simulink model "nosaturation"  (R2016b)
settings: Solver=VariableStepAuto  StartTime=0.0  StopTime=48*60  RelTol=1e-3
values from neighbouring files (symbols this model uses):
  d1 = i_den(1)    [Qdesign.m]    (also in Qdesign2.m)
  d2 = i_den(2)    [Qdesign.m]    (also in Qdesign2.m)
  d3 = i_den(3)    [Qdesign.m]    (also in Qdesign2.m)
  d4 = i_den(4)    [Qdesign.m]    (also in Qdesign2.m)
  Ki = -0.075    [defineparams.m]    (also in smithpredictor_1.m)
  Km = 4    [defineparams.m]    (also in smithpredictor_1.m)
  n1 = 0    [Qdesign.m]    (also in Qdesign2.m)
  n2 = i_num(1)    [Qdesign.m]    (also in Qdesign2.m)
  n3 = i_num(2)    [Qdesign.m]    (also in Qdesign2.m)
  n4 = i_num(3)    [Qdesign.m]    (also in Qdesign2.m)
  s_den = double(coeffs(Q_simple_den))    [Qdesign.m]    (also in Qdesign2.m)
  s_num = [0 double(coeffs(Q_simple_num))]    [Qdesign.m]    (also in Qdesign2.m)
  Tdi = 25    [defineparams.m]    (also in smithpredictor_1.m)
  Tdm = 15    [defineparams.m]    (also in smithpredictor_1.m)
  Ti = 140    [defineparams.m]    (also in smithpredictor_1.m)
  Tm = 50    [defineparams.m]    (also in smithpredictor_1.m)
settings Model: Creator=Matt Cordoba  LastModifiedBy=Matt Cordoba

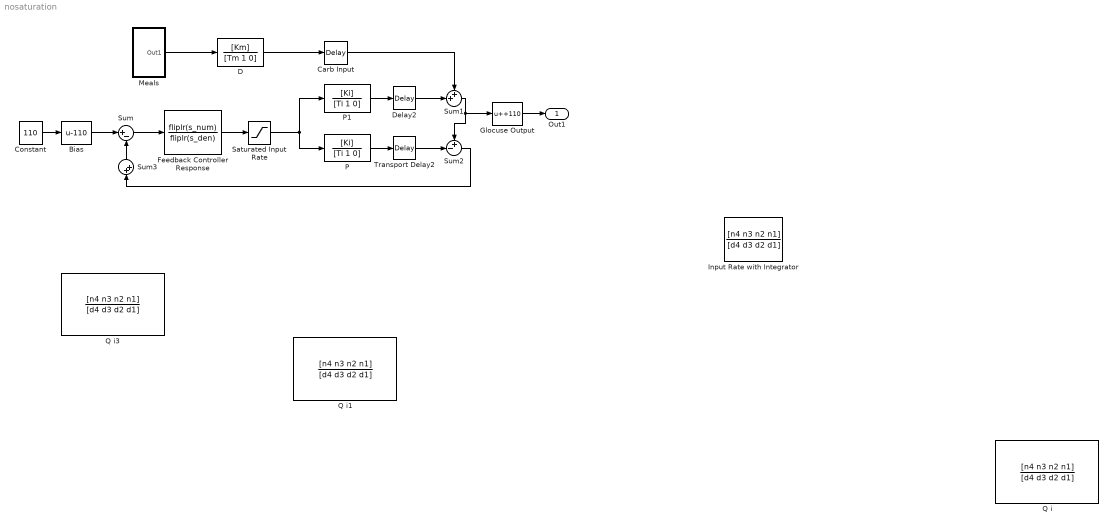
== system nosaturation ==
  Bias : Bias  Bias=-110
  Carb Input : TransportDelay  DelayTime=Tdm
  Constant : Constant  Value=110
  D : TransferFcn  Numerator=[Km]  Denominator=[Tm 1 0]
  Delay2 : TransportDelay  DelayTime=Tdi
  Feedback Controller Response : TransferFcn  Numerator=fliplr(s_num)  Denominator=fliplr(s_den)
  Glocuse Output : Bias  Bias=+110
  Input Rate with Integrator : TransferFcn  Numerator=[n4 n3 n2 n1]  Denominator=[d4 d3 d2 d1]
  Meals : Subsystem
  P : TransferFcn  Numerator=[Ki]  Denominator=[Ti 1 0]
  P1 : TransferFcn  Numerator=[Ki]  Denominator=[Ti 1 0]
  Q i : TransferFcn  Numerator=[n4 n3 n2 n1]  Denominator=[d4 d3 d2 d1]
  Q i1 : TransferFcn  Numerator=[n4 n3 n2 n1]  Denominator=[d4 d3 d2 d1]
  Q i3 : TransferFcn  Numerator=[n4 n3 n2 n1]  Denominator=[d4 d3 d2 d1]
  Saturated Input Rate : Saturate  UpperLimit=166  LowerLimit=0
  Sum : Sum  Inputs=|+-
  Sum1 : Sum  Inputs=++|
  Sum2 : Sum  Inputs=+-|
  Sum3 : Sum  Inputs=|++
  Transport Delay2 : TransportDelay  DelayTime=Tdi
  Out1 : Outport
  wires:
  D/1 -> Carb Input/1
  P/1 -> Transport Delay2/1
  Carb Input/1 -> Sum1/1
  P1/1 -> Delay2/1
  Delay2/1 -> Sum1/2
  Transport Delay2/1 -> Sum2/2
  Sum2/1 -> Sum3/1
  Sum3/1 -> Sum/2
  Meals/1(Out1) -> D/1
  Constant/1 -> Bias/1
  Bias/1 -> Sum/1
  Sum1/1 -> Glocuse Output/1, Sum2/1
  Glocuse Output/1 -> Out1/1
  Sum/1 -> Feedback Controller Response/1
  Feedback Controller Response/1 -> Saturated Input Rate/1
  Saturated Input Rate/1 -> P1/1, P/1

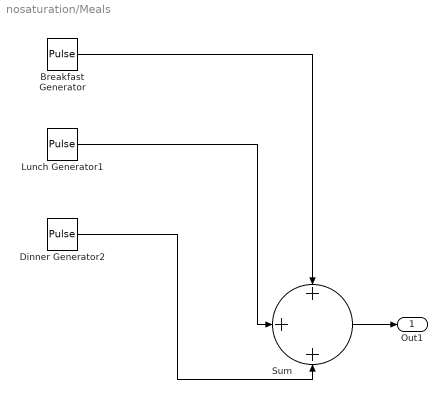
== system nosaturation/Meals ==
  Breakfast Generator : DiscretePulseGenerator  Amplitude=25/10  Period=1440  PulseWidth=10  PhaseDelay=60
  Dinner Generator2 : DiscretePulseGenerator  Amplitude=3  Period=1440  PulseWidth=20  PhaseDelay=540
  Lunch Generator1 : DiscretePulseGenerator  Amplitude=40/15  Period=1440  PulseWidth=15  PhaseDelay=420
  Sum : Sum  Inputs=+++
  Out1 : Outport
  wires:
  Breakfast Generator/1 -> Sum/1
  Lunch Generator1/1 -> Sum/2
  Dinner Generator2/1 -> Sum/3
  Sum/1 -> Out1/1
